simulink model "AEMACE_ECU"  (R2021b)
settings: Solver=FixedStepDiscrete  StartTime=0.0  StopTime=inf  RelTol=1e-3
undefined symbols (not defined in the file or in its folder): AEMACE8_AECU8_ACTUATOR_SPEED_CMD, AEMACE8_AECU8_BRAKE_CMD_AWARENESS, AEMACE8_AECU8_DELTAP_FAILURE, AEMACE8_AECU8_HB, AEMACE8_AECU8_OPERATIONAL_MODE_CMD, AEMACE8_AECU8_WOW1, AEMACE8_AECU8_WOW2, IO682
libraries: speedgoatlib_IO682 x3
settings Model: Creator=ACH  LastModifiedBy=angel
settings SolverCC: ConcurrentTasks=on  PositivePriorityOrder=on
settings OptimizationCC: BlockReduction=off  OptimizeBlockIOStorage=off
settings DebuggingCC: TasksWithSamePriorityMsg=none
settings HardwareCC: ProdBitPerLong=64  ProdLongLongMode=on  ProdHWDeviceType=Intel->x86-64 (Linux 64)
settings RTWCC: Description=Simulink Real-Time  SystemTargetFile=slrealtime.tlc  TemplateMakefile=slrealtime_default_tmf  Toolchain=Simulink Real-Time Toolchain  BuildConfiguration=Faster Runs  CodeExecutionProfiling=on  TargetLang=C++
settings SimulinkRealTimeTargetCC: UseGCCFastMath=on

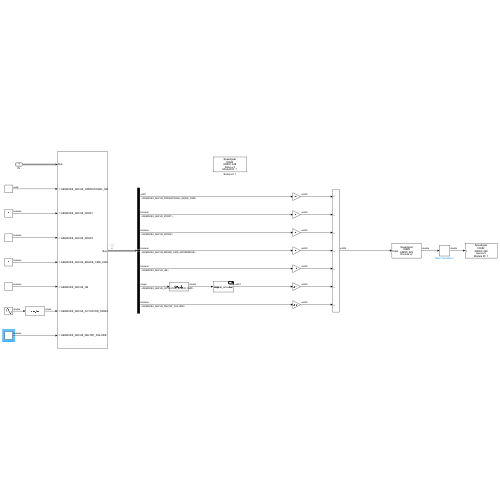
[thumbnail: Simulink's stored preview of the top-level diagram]
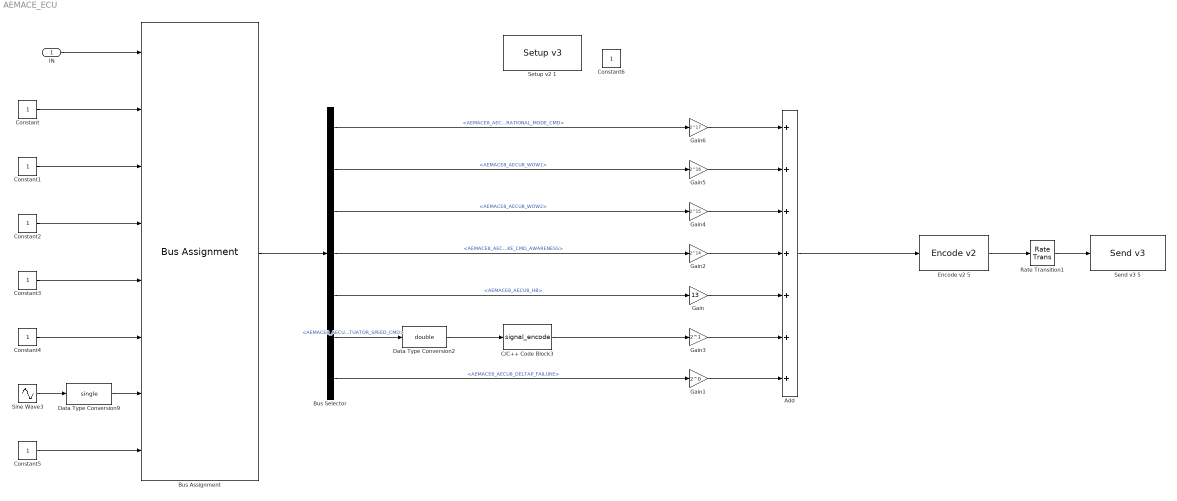
== system AEMACE_ECU ==
  IN : Inport  OutDataTypeStr=Bus: AEMACE8_AECU8_1
  Add : Sum  Inputs=+++++++
  Bus Assignment : BusAssignment  AssignedSignals=AEMACE8_AECU8_OPERATIONAL_MODE_CMD,AEMACE8_AECU8_WOW1,AEMACE8_AECU8_WOW2,AEMACE8_AECU8_BRAKE_CMD_AWARENESS,AEMACE8_AECU8_HB,AEMACE8_AECU8_ACTUATOR_SPEED_CMD,AEMACE8_AECU8_DELTAP_FAILURE
  Bus Selector : BusSelector  OutputSignals=AEMACE8_AECU8_OPERATIONAL_MODE_CMD,AEMACE8_AECU8_WOW1,AEMACE8_AECU8_WOW2,AEMACE8_AECU8_BRAKE_CMD_AWARENESS,AEMACE8_AECU8_HB,AEMACE8_AECU8_ACTUATOR_SPEED_CMD,AEMACE8_AECU8_DELTAP_FAILURE
  C/C++ Code Block3 : S-Function  FunctionName=signal_encode  Parameters=5/128,0,boolean(1),boolean(0),uint32(12)  SFunctionModules=signal_encode_wrapper  SFunctionDeploymentMode=off  EnableBusSupport=off  mask(S-Function Builder){}
      mask help: Simulink:masks:SFunctionBuilder_MD
      mask init:
      | val = [[.9  0.75 0.75 1 1 .9 .9 1]',[1 1 0.75 0.75 .9 .9 1 .9]'];try , sys = get_param(gcb,'SfunBuilderFcnName');if isempty(sys), sys = get_param(gcb,'FunctionName'); end,catch, sys = get_param(gcb,'FunctionName'); end
      settings: CopyFcn=set_param(gcbh,'LinkStatus','none')  OpenFcn=sfunctionwizard(gcbh)
      mask Display:
      | plot(val(:,1),val(:,2))
      | disp(sys)
      | port_label('input',1,'data')
      | port_label('output',1,'out')
  Constant : Constant  OutDataTypeStr=uint8
  Constant{1..5} (5 alike) : Constant  OutDataTypeStr=boolean
  Data Type Conversion2 : DataTypeConversion  OutDataTypeStr=double
  Data Type Conversion9 : DataTypeConversion  OutDataTypeStr=single
  Encode v2 5 : speedgoatlib_IO682/Encode v2   parMode=Custom Data Type  parLabel=[231]  parDataType=[0]  parResolution=[1]  parBits=[19]  parSdi=[0]  parSsm=[-1]  parCustomDataType=Raw  parDataLSB=11  parDataMSB=31  parBitPosition=[9, 31]  parScaleBNR=1  parExponent=8  parMantissa=14  parEnSSM=off
      settings: SourceProductName=Simulink Real-Time: Speedgoat I/O Blockset
  Gain : Gain  Gain=13  OutDataTypeStr=uint32
  Gain1 : Gain  Gain=2^0  OutDataTypeStr=uint32
  Gain2 : Gain  Gain=2^14  OutDataTypeStr=uint32
  Gain3 : Gain  Gain=2^1  OutDataTypeStr=uint32
  Gain4 : Gain  Gain=2^15  OutDataTypeStr=uint32
  Gain5 : Gain  Gain=2^16  OutDataTypeStr=uint32
  Gain6 : Gain  Gain=2^17  OutDataTypeStr=uint32
  Rate Transition1 : RateTransition
  Send v3 5 : speedgoatlib_IO682/Send v3   parModuleId=1  parChannel=1  parSampleTime=0.008
      settings: SourceProductName=Simulink Real-Time: Speedgoat I/O Blockset
  Setup v2 1 : speedgoatlib_IO682/Setup v3   parModuleId=1  parBoardVariant=IO682-16-16  parPciSlot=-1  parTimerCount=4000*8  parChannelMode=Manual  parInBitRate1=100000  parInBufferMode1=Individual  parInEnable1=on  parInParity1=off  parInInternalWrap1=off  parInBitRate2=100000  parInBufferMode2=Individual  parInEnable2=on  parInParity2=on  parInInternalWrap2=off  parInBitRate3=100000  parInBufferMode3=Individual  parInEnable3=on  parInParity3=on  parInInternalWrap3=off  parInBitRate4=100000  parInBufferMode4=Individual  parInEnable4=on  parInParity4=on  parInInternalWrap4=off  parInBitRate5=100000  parInBufferMode5=Individual  parInEnable5=on  parInParity5=on  parInInternalWrap5=off  parInBitRate6=100000  parInBufferMode6=Individual  parInEnable6=on  parInParity6=on  parInInternalWrap6=off  parInBitRate7=100000  parInBufferMode7=Individual  parInEnable7=on  parInParity7=on  parInInternalWrap7=off  parInBitRate8=100000  parInBufferMode8=Individual  parInEnable8=on  parInParity8=on  parInInternalWrap8=off  parInBitRate9=100000  parInBufferMode9=Individual  parInEnable9=on  parInParity9=on  parInInternalWrap9=off  parInBitRate10=100000  parInBufferMode10=Individual  parInEnable10=on  parInParity10=on  parInInternalWrap10=off  parInBitRate11=100000  parInBufferMode11=Individual  parInEnable11=on  parInParity11=on  parInInternalWrap11=off  parInBitRate12=100000  parInBufferMode12=Individual  parInEnable12=on  parInParity12=on  parInInternalWrap12=off  parInBitRate13=100000  parInBufferMode13=Individual  parInEnable13=on  parInParity13=on  parInInternalWrap13=off  parInBitRate14=100000  parInBufferMode14=Individual  parInEnable14=on  parInParity14=on  parInInternalWrap14=off  parInBitRate15=100000  parInBufferMode15=Individual  parInEnable15=on  parInParity15=on  parInInternalWrap15=off  parInBitRate16=100000  parInBufferMode16=Individual  parInEnable16=on  parInParity16=on  parInInternalWrap16=off  parOutBitRate1=100000  parOutParity1=Odd  parOutProtocolError1=None  parOutEnable1=on  parOutBitRate2=100000  parOutParity2=Odd  parOutProtocolError2=None  parOutEnable2=on  parOutBitRate3=100000  parOutParity3=Odd  parOutProtocolError3=None  parOutEnable3=on  parOutBitRate4=100000  parOutParity4=Odd  parOutProtocolError4=None  parOutEnable4=on  parOutBitRate5=100000  parOutParity5=Odd  parOutProtocolError5=None  parOutEnable5=on  parOutBitRate6=100000  parOutParity6=Odd  parOutProtocolError6=None  parOutEnable6=on  parOutBitRate7=100000  parOutParity7=Odd  parOutProtocolError7=None  parOutEnable7=on  parOutBitRate8=100000  parOutParity8=Odd  parOutProtocolError8=None  parOutEnable8=on  parOutBitRate9=100000  parOutParity9=Odd  parOutProtocolError9=None  parOutEnable9=on  parOutBitRate10=100000  parOutParity10=Odd  parOutProtocolError10=None  parOutEnable10=on  parOutBitRate11=100000  parOutParity11=Odd  parOutProtocolError11=None  parOutEnable11=on  parOutBitRate12=100000  parOutParity12=Odd  parOutProtocolError12=None  parOutEnable12=on  parOutBitRate13=100000  parOutParity13=Odd  parOutProtocolError13=None  parOutEnable13=on  parOutBitRate14=100000  parOutParity14=Odd  parOutProtocolError14=None  parOutEnable14=on  parOutBitRate15=100000  parOutParity15=Odd  parOutProtocolError15=None  parOutEnable15=on  parOutBitRate16=100000  parOutParity16=Odd  parOutProtocolError16=None  parOutEnable16=on  parChConfigFile=''  parScheduleMode=Manual  parScheduledMsgConfigFile=''  parHwDeviceId=hex2dec('0830')  parTimeSource=Internal timer  parChInConfig=[158 8 7 8 1;158 8 7 7 1;158 8 7 7 1;158 8 7 7 1;158 8 7 7 1;158 8 7 7 1;158 8 7 7 1;158 8 7 7 1;158 8 7 7 1;158 8 7 7 1;158 8 7 7 1;158 8 7 7 1;158 8 7 7 1;158 8 7 7 1;158 8 7 7 1;158 8 7 7 1]  parChOutConfig=[158 0 4 7;158 0 4 7;158 0 4 7;158 0 4 7;158 0 4 7;158 0 4 7;158 0 4 7;158 0 4 7;158 0 4 7;158 0 4 7;158 0 4 7;158 0 4 7;158 0 4 7;158 0 4 7;158 0 4 7;158 0 4 7]  parScheduledMessages=0
      settings: SourceProductName=Speedgoat I/O Blockset
  Sine Wave3 : Sin  Amplitude=80*0.99  Frequency=2*pi  SampleTime=0.008
  Constant6 : Constant  IOType=siggen
  wires:
  Encode v2 5/1 -> Rate Transition1/1
  Add/1 -> Encode v2 5/1
  Bus Assignment/1 -> Bus Selector/1
  Gain2/1 -> Add/4
  Gain/1 -> Add/5
  Gain3/1 -> Add/6
  Gain1/1 -> Add/7
  IN/1 -> Bus Assignment/1
  Data Type Conversion2/1 -> C/C++ Code Block3/1
  Rate Transition1/1 -> Send v3 5/1
  Bus Selector/7 -> Gain1/1  "<AEMACE8_AECU8_DELTAP_FAILURE>"
  Bus Selector/6 -> Data Type Conversion2/1  "<AEMACE8_AECU8_ACTUATOR_SPEED_CMD>"
  C/C++ Code Block3/1 -> Gain3/1
  Bus Selector/5 -> Gain/1  "<AEMACE8_AECU8_HB>"
  Bus Selector/4 -> Gain2/1  "<AEMACE8_AECU8_BRAKE_CMD_AWARENESS>"
  Gain4/1 -> Add/3
  Bus Selector/3 -> Gain4/1  "<AEMACE8_AECU8_WOW2>"
  Bus Selector/2 -> Gain5/1  "<AEMACE8_AECU8_WOW1>"
  Gain5/1 -> Add/2
  Gain6/1 -> Add/1
  Bus Selector/1 -> Gain6/1  "<AEMACE8_AECU8_OPERATIONAL_MODE_CMD>"
  Constant/1 -> Bus Assignment/2
  Constant2/1 -> Bus Assignment/4
  Constant1/1 -> Bus Assignment/3
  Constant3/1 -> Bus Assignment/5
  Constant4/1 -> Bus Assignment/6
  Constant5/1 -> Bus Assignment/8
  Data Type Conversion9/1 -> Bus Assignment/7
  Sine Wave3/1 -> Data Type Conversion9/1
